simulink library "lib_controller"  (R2015a)
settings: Solver=ode45  StartTime=0.0  StopTime=10.0  RelTol=1e-3
values from neighbouring files (symbols this model uses):
  CG_0 = [0,0,0.02]'    [SetupComplete.m]
  g = 9.81    [SetupComplete.m]
  h_M = 0.064    [SetupComplete.m]
  I_BAC_0 = [ Ix,0,Ixz;0,Iy,0;Ixz,0,Iz]    [SetupComplete.m]
  l = 0.3450    (= 0.345)    [NDI_components.m]    (also in SetupComplete.m; robust_controller.m)
  m = 3.51    [SetupComplete.m]
  m_0 = 2.61    [SetupComplete.m]
  m_M = 0.300    (= 0.3)    [SetupComplete.m]
  T_sim = 0.01    [Run3Copter.m]
undefined symbols (not defined in the file or in its folder): Theta_1_roll_last, Theta_2_roll_last, Theta_3_roll_last, V_long_lastA_w_z, V_long_lastAoA, V_roll_last, V_yaw_last, W_long_lastA_w_z, W_long_lastAoA, W_roll_last, W_yaw_last
libraries: simulink x65, Adaptive_FaultTolerantControl x8, lib_controller x5, qcatlib x4, dspinverses x4, aerolibtransform2 x3, aerolib6dofsys x1
(part 1 of 10)
settings Model: Creator=juan  LastModifiedBy=juan

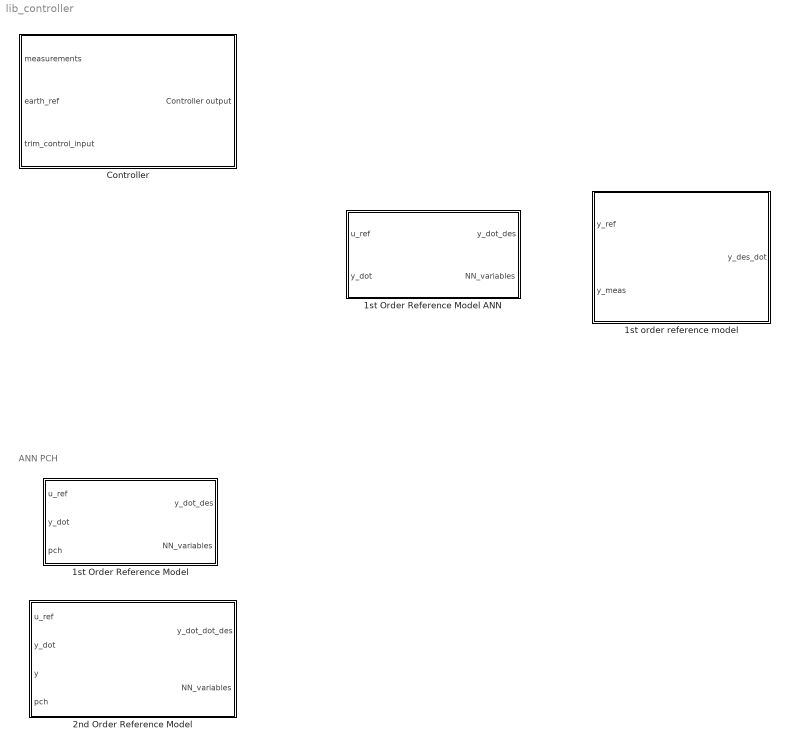
== system lib_controller ==
  note: ANN PCH
  1st Order Reference Model : Subsystem  mask{tau=0.25, r=1}
      mask prompts: tau "Time Constant"; r "NN Error dynamic ratio"
      mask help:
      | 1st Order Model Reference System
      | Tau is the time constant and sets the dynamics of the reference model.
      | Error dynamic ratio sets how faster compared to the reference model is the
      | NN output going to try to compensate for the inversion error.
      mask Display:
      | K_ref=1/tau;
      | TF = tf([K_ref],[1 K_ref]);
      | 
      | [y,t]=step(TF);
      | S = stepinfo(y,t);
      | 
      | pos = get_param(gcb, 'Position');
      | width = pos(3) - pos(1);
      | height = pos(4) - pos(2);
      | t = t.*width/max(t);
      | y=y.*height/max(y);
      | plot(t,y);
      | S2 = stepinfo(y,t);
      | 
      | if S.Overshoot==0 % 1st order response
      |     text(S2.RiseTime ,height*0.85,['Rise time = ',num2str(S.RiseTime),'s' ]);
      |     text(S2.RiseTime ,height*0.75,['Settling Time = ',num2str(S.SettlingTime)]);
      | 
      | elseif S.Overshoot<0.05 % 2nd order response
      |     text(width*0.5 ,height*0.9,['Rise time = ',num2str(S.RiseTime),'s' ]);
      |     text(width*0.5 ,height*0.8,['Pike time = ',num2str(S.PeakTime),'s' ]);
      |     text(width*0.5 ,height*0.7,['Os = ',num2str(S.Peak)]);
      |     text(width*0.5 ,height*0.6,['SettlingTime = ',num2str(S.SettlingTime)]);
      | else % 2nd order response
      |     text(S2.PeakTime ,S2.Peak*0.85,['Peak time = ',num2str(S.PeakTime),'s' ]);
      |     text(S2.PeakTime ,S2.Peak*0.75,['Os = ',num2str(S.Peak)]);
      |     text(S2.PeakTime ,S2.Peak*0.65,['SettlingTime = ',num2str(S.SettlingTime)]);
      | end
      | 
      | 
      | [num,den] = tfdata(TF);
      | dpoly(num{:},den{:}, 's');
  1st Order Reference Model ANN : Subsystem  mask{tau=0.25, r=1}
      mask prompts: tau "Time Constant"; r "NN Error dynamic ratio"
      mask help:
      | 1st Order Model Reference System
      | Tau is the time constant and sets the dynamics of the reference model.
      | Error dynamic ratio sets how faster compared to the reference model is the
      | NN output going to try to compensate for the inversion error.
      mask Display:
      | K_ref=1/tau;
      | TF = tf([K_ref],[1 K_ref]);
      | 
      | [y,t]=step(TF);
      | S = stepinfo(y,t);
      | 
      | pos = get_param(gcb, 'Position');
      | width = pos(3) - pos(1);
      | height = pos(4) - pos(2);
      | t = t.*width/max(t);
      | y=y.*height/max(y);
      | plot(t,y);
      | S2 = stepinfo(y,t);
      | 
      | if S.Overshoot==0 % 1st order response
      |     text(S2.RiseTime ,height*0.85,['Rise time = ',num2str(S.RiseTime),'s' ]);
      |     text(S2.RiseTime ,height*0.75,['Settling Time = ',num2str(S.SettlingTime)]);
      | 
      | elseif S.Overshoot<0.05 % 2nd order response
      |     text(width*0.5 ,height*0.9,['Rise time = ',num2str(S.RiseTime),'s' ]);
      |     text(width*0.5 ,height*0.8,['Pike time = ',num2str(S.PeakTime),'s' ]);
      |     text(width*0.5 ,height*0.7,['Os = ',num2str(S.Peak)]);
      |     text(width*0.5 ,height*0.6,['SettlingTime = ',num2str(S.SettlingTime)]);
      | else % 2nd order response
      |     text(S2.PeakTime ,S2.Peak*0.85,['Peak time = ',num2str(S.PeakTime),'s' ]);
      |     text(S2.PeakTime ,S2.Peak*0.75,['Os = ',num2str(S.Peak)]);
      |     text(S2.PeakTime ,S2.Peak*0.65,['SettlingTime = ',num2str(S.SettlingTime)]);
      | end
      | 
      | 
      | [num,den] = tfdata(TF);
      | dpoly(num{:},den{:}, 's');
  1st order reference model : Subsystem  mask(1st order model reference block){Kref=10, Kb=10, fi=0.25, fc=0.5, Kf=1}
      mask prompts: Kref "1st order reference gain"; Kb "Bandwidth gain"; fi "Integral gain"; fc "Command FF gain"; Kf "Command_dot FF gain"
      mask help:
      | Generates a desired first order derivative of a commanded output taking
      | into account the current measured output.
      | Kref is the gain that determines the first order system between y_ref and
      | y_commanded signals. Ycom/Yref = Kref/(1 + Kref)
      | fi and fc can be defaulted to 0.25 and 0.5 for a critically damped 2nd
      | order response between y_meas and the error signal (y_com - y_meas) considering
      | a perfect dynamic inversion.
      mask Help:
      | Juan Herrero Macias <jn.herrerom@gmail.com>
      | This architecture can be found and explained in Fault-tolerant Flight
      | Control and Guidance Systems, Ducard, Guillaume.
      mask TypeOptions Kref: Kref gain/Gain
      mask TypeOptions Kb: Bandwidth gain/Gain
      mask TypeOptions fi: Integral gain/Gain
      mask TypeOptions fc: Command FF gain/Gain
      mask TypeOptions Kf: Command_dot FF gain/Gain
  2nd Order Reference Model : Subsystem  mask{omega_n=4, xi=1.1, r=0}
      mask prompts: omega_n "Natural Frequency"; xi "Damping"; r "NN Error dynamic ratio"
      mask help:
      | 2nd Order Model Reference System
      | Natural frequency and damping ratio set the dynamic of the model reference.
      | Error dynamic ratio sets how faster compared to the reference model dynamics
      | is the settling time of the inversion error provided by the NN.
      mask Display:
      | TF = tf([omega_n^2],[1 2*xi*omega_n omega_n^2]);
      | 
      | [y,t]=step(TF);
      | S = stepinfo(y,t);
      | 
      | pos = get_param(gcb, 'Position');
      | width = pos(3) - pos(1);
      | height = pos(4) - pos(2);
      | t = t.*width/max(t);
      | y=y.*height/max(y);
      | plot(t,y);
      | S2 = stepinfo(y,t);
      | 
      | if S.Overshoot==0 % 1st order response
      |     text(S2.RiseTime ,height*0.85,['Rise time = ',num2str(S.RiseTime),'s' ]);
      |     text(S2.RiseTime ,height*0.75,['Settling Time = ',num2str(S.SettlingTime)]);
      | 
      | elseif S.Overshoot<0.05 % 2nd order response
      |     text(width*0.5 ,height*0.9,['Rise time = ',num2str(S.RiseTime),'s' ]);
      |     text(width*0.5 ,height*0.8,['Pike time = ',num2str(S.PeakTime),'s' ]);
      |     text(width*0.5 ,height*0.7,['Os = ',num2str(S.Peak)]);
      |     text(width*0.5 ,height*0.6,['SettlingTime = ',num2str(S.SettlingTime)]);
      | else % 2nd order response
      |     text(S2.PeakTime ,S2.Peak*0.85,['Peak time = ',num2str(S.PeakTime),'s' ]);
      |     text(S2.PeakTime ,S2.Peak*0.75,['Os = ',num2str(S.Peak)]);
      |     text(S2.PeakTime ,S2.Peak*0.65,['SettlingTime = ',num2str(S.SettlingTime)]);
      | end
      | 
      | 
      | [num,den] = tfdata(TF);
      | dpoly(num{:},den{:}, 's');
  Controller : Subsystem  Variant=on  OverrideUsingVariant=Variant1

== system lib_controller/1st Order Reference Model ==
  u_ref : Inport
  y_dot : Inport  Port=2
  pch : Inport  Port=3
  A_error_dynamics : Constant  Value=-r/tau
  Bus Creator : BusCreator  Inputs=6
  Kp_y : Gain  Gain=r/tau
  P_error_dynamics : Constant  Value=tau/r
  Reference Model : Subsystem  mask{tau=tau, y_i=0}
      mask prompts: tau "1st order time constant (tau)"; y_i "Initial state"
      mask init:
      | K_ref=1/tau;
      mask Display:
      | K_ref=1/tau;
      | TF = tf([K_ref],[1 K_ref]);
      | 
      | [y,t]=step(TF);
      | S = stepinfo(y,t);
      | 
      | pos = get_param(gcb, 'Position');
      | width = pos(3) - pos(1);
      | height = pos(4) - pos(2);
      | t = t.*width/max(t);
      | y=y.*height/max(y);
      | plot(t,y);
      | S2 = stepinfo(y,t);
      | 
      | if S.Overshoot==0 % 1st order response
      |     text(S2.RiseTime ,height*0.85,['Rise time = ',num2str(S.RiseTime),'s' ]);
      |     text(S2.RiseTime ,height*0.75,['Settling Time = ',num2str(S.SettlingTime)]);
      | 
      | elseif S.Overshoot<0.05 % 2nd order response
      |     text(width*0.5 ,height*0.9,['Rise time = ',num2str(S.RiseTime),'s' ]);
      |     text(width*0.5 ,height*0.8,['Pike time = ',num2str(S.PeakTime),'s' ]);
      |     text(width*0.5 ,height*0.7,['Os = ',num2str(S.Peak)]);
      |     text(width*0.5 ,height*0.6,['SettlingTime = ',num2str(S.SettlingTime)]);
      | else % 2nd order response
      |     text(S2.PeakTime ,S2.Peak*0.85,['Peak time = ',num2str(S.PeakTime),'s' ]);
      |     text(S2.PeakTime ,S2.Peak*0.75,['Os = ',num2str(S.Peak)]);
      |     text(S2.PeakTime ,S2.Peak*0.65,['SettlingTime = ',num2str(S.SettlingTime)]);
      | end
      | 
      | 
      | [num,den] = tfdata(TF);
      | dpoly(num{:},den{:}, 's');
  Sum17 : Sum  Inputs=++|
  Sum22 : Sum  Inputs=|+-
  b_error_dynamics : Constant  Value=[1]  VectorParams1D=off
  y_dot_des : Outport
  NN_variables : Outport  Port=2
  wires:
  u_ref/1 -> Reference Model/1(u)
  Reference Model/2(y) -> Bus Creator/2, Sum22/1  "y_c"
  Reference Model/1(y_dot) -> Bus Creator/3, Sum17/1  "y_dot_c"
  y_dot/1 -> Sum22/2
  Sum22/1 -> Bus Creator/1, Kp_y/1  "y_error"
  Kp_y/1 -> Sum17/2
  Sum17/1 -> y_dot_des/1
  Bus Creator/1 -> NN_variables/1
  A_error_dynamics/1 -> Bus Creator/5  "A_error_dyn"
  P_error_dynamics/1 -> Bus Creator/4  "P_error_dyn"
  b_error_dynamics/1 -> Bus Creator/6  "b_error_dyn"
  pch/1 -> Reference Model/2(pch)

== system lib_controller/1st Order Reference Model ANN ==
  u_ref : Inport
  y_dot : Inport  Port=2
  A_error_dynamics : Constant  Value=-r/tau
  Bus Creator : BusCreator  Inputs=6
  Kp_y : Gain  Gain=r/tau
  P_error_dynamics : Constant  Value=tau/r
  Reference Model : Subsystem  mask{tau=tau, y_i=0}
      mask prompts: tau "1st order time constant (tau)"; y_i "Initial state"
      mask init:
      | K_ref=1/tau;
      mask Display:
      | K_ref=1/tau;
      | TF = tf([K_ref],[1 K_ref]);
      | 
      | [y,t]=step(TF);
      | S = stepinfo(y,t);
      | 
      | pos = get_param(gcb, 'Position');
      | width = pos(3) - pos(1);
      | height = pos(4) - pos(2);
      | t = t.*width/max(t);
      | y=y.*height/max(y);
      | plot(t,y);
      | S2 = stepinfo(y,t);
      | 
      | if S.Overshoot==0 % 1st order response
      |     text(S2.RiseTime ,height*0.85,['Rise time = ',num2str(S.RiseTime),'s' ]);
      |     text(S2.RiseTime ,height*0.75,['Settling Time = ',num2str(S.SettlingTime)]);
      | 
      | elseif S.Overshoot<0.05 % 2nd order response
      |     text(width*0.5 ,height*0.9,['Rise time = ',num2str(S.RiseTime),'s' ]);
      |     text(width*0.5 ,height*0.8,['Pike time = ',num2str(S.PeakTime),'s' ]);
      |     text(width*0.5 ,height*0.7,['Os = ',num2str(S.Peak)]);
      |     text(width*0.5 ,height*0.6,['SettlingTime = ',num2str(S.SettlingTime)]);
      | else % 2nd order response
      |     text(S2.PeakTime ,S2.Peak*0.85,['Peak time = ',num2str(S.PeakTime),'s' ]);
      |     text(S2.PeakTime ,S2.Peak*0.75,['Os = ',num2str(S.Peak)]);
      |     text(S2.PeakTime ,S2.Peak*0.65,['SettlingTime = ',num2str(S.SettlingTime)]);
      | end
      | 
      | 
      | [num,den] = tfdata(TF);
      | dpoly(num{:},den{:}, 's');
  Sum17 : Sum  Inputs=++|
  Sum22 : Sum  Inputs=|+-
  b_error_dynamics : Constant  Value=[1]  VectorParams1D=off
  y_dot_des : Outport
  NN_variables : Outport  Port=2
  wires:
  b_error_dynamics/1 -> Bus Creator/6  "b_error_dyn"
  P_error_dynamics/1 -> Bus Creator/4  "P_error_dyn"
  A_error_dynamics/1 -> Bus Creator/5  "A_error_dyn"
  Bus Creator/1 -> NN_variables/1
  Sum17/1 -> y_dot_des/1
  Kp_y/1 -> Sum17/2
  Sum22/1 -> Kp_y/1, Bus Creator/1  "y_error"
  y_dot/1 -> Sum22/2
  Reference Model/1(y_dot) -> Sum17/1, Bus Creator/3  "y_dot_c"
  Reference Model/2(y) -> Sum22/1, Bus Creator/2  "y_c"
  u_ref/1 -> Reference Model/1(u)

== system lib_controller/1st order reference model ==
  y_ref : Inport
  y_meas : Inport  Port=2
  Bandwidth gain : Gain  Gain=Kb
  Bandwidth gain 1 : Gain  Gain=Kb
  Command FF gain : Gain  Gain=fc
  Command_dot FF gain : Gain  Gain=Kf
  Integral gain : Gain  Gain=fi
  Integrator : Integrator
  Integrator1 : Integrator
  Kref gain : Gain  Gain=Kref
  Sum15 : Sum  Inputs=|+-
  Sum16 : Sum  Inputs=++-
  Sum17 : Sum  Inputs=++|
  Sum5 : Sum  Inputs=|+-
  y_des_dot : Outport
  wires:
  Sum5/1 -> Kref gain/1
  Sum15/1 -> Bandwidth gain 1/1
  Bandwidth gain/1 -> Sum17/2
  Sum17/1 -> y_des_dot/1
  Integrator1/1 -> Sum16/2
  Kref gain/1 -> Command_dot FF gain/1, Integrator/1  "y_dot_c"
  Sum16/1 -> Bandwidth gain/1
  y_meas/1 -> Sum15/2, Sum16/3
  Integrator/1 -> Sum5/2, Sum15/1, Command FF gain/1  "y_c"
  Command FF gain/1 -> Sum16/1
  Command_dot FF gain/1 -> Sum17/1
  y_ref/1 -> Sum5/1
  Bandwidth gain 1/1 -> Integral gain/1
  Integral gain/1 -> Integrator1/1

== system lib_controller/2nd Order Reference Model ==
  u_ref : Inport
  y_dot : Inport  Port=2
  y : Inport  Port=3
  pch : Inport  Port=4
  A_error_dynamics1 : Constant  Value=[0, 1; -(r*omega_n)^2, -2*xi*(r*omega_n)]
  Bus Creator : BusCreator  Inputs=8
  Kd_y_dot : Gain  Gain=2*xi*(r*omega_n)
  Kp_y : Gain  Gain=(r*omega_n)^2
  P_error_dynamics1 : Constant  Value=[((r*omega_n)^2+1)/(2*xi*(r*omega_n)) + 2*xi*(r*omega_n)/(r*omega_n)^2, 1/(r*omega_n)^2; 1/(r*omega_n)^2, (1+1/(r*omega_n)^2)/(2*xi*(r*omega_n))]
  Reference Model1 : Subsystem  mask{omega_n=omega_n, xi=xi}
      mask prompts: omega_n "Natural Frequency"; xi "Damping"
      mask help:
      | 2nd Order System
      | Only provides output acceleration
      mask Display:
      | TF = tf([omega_n^2],[1 xi*omega_n omega_n^2]);
      | 
      | [y,t]=step(TF);
      | S = stepinfo(y,t);
      | 
      | pos = get_param(gcb, 'Position');
      | width = pos(3) - pos(1);
      | height = pos(4) - pos(2);
      | t = t.*width/max(t);
      | y=y.*height/max(y);
      | plot(t,y);
      | S2 = stepinfo(y,t);
      | 
      | if S.Overshoot==0 % 1st order response
      |     text(S2.RiseTime ,height*0.85,['Rise time = ',num2str(S.RiseTime),'s' ]);
      |     text(S2.RiseTime ,height*0.75,['Settling Time = ',num2str(S.SettlingTime)]);
      | 
      | elseif S.Overshoot<0.05 % 2nd order response
      |     text(width*0.5 ,height*0.9,['Rise time = ',num2str(S.RiseTime),'s' ]);
      |     text(width*0.5 ,height*0.8,['Pike time = ',num2str(S.PeakTime),'s' ]);
      |     text(width*0.5 ,height*0.7,['Os = ',num2str(S.Peak)]);
      |     text(width*0.5 ,height*0.6,['SettlingTime = ',num2str(S.SettlingTime)]);
      | else % 2nd order response
      |     text(S2.PeakTime ,S2.Peak*0.85,['Peak time = ',num2str(S.PeakTime),'s' ]);
      |     text(S2.PeakTime ,S2.Peak*0.75,['Os = ',num2str(S.Peak)]);
      |     text(S2.PeakTime ,S2.Peak*0.65,['SettlingTime = ',num2str(S.SettlingTime)]);
      | end
      | 
      | 
      | [num,den] = tfdata(TF);
      | dpoly(num{:},den{:}, 's');
  Sum19 : Sum  Inputs=|+-
  Sum20 : Sum  Inputs=+++
  Sum21 : Sum  Inputs=|+-
  b_error_dynamics : Constant  Value=[0; 1]  VectorParams1D=off
  y_dot_dot_des : Outport
  NN_variables : Outport  Port=2
  wires:
  Reference Model1/1(y_dot_dot) -> Bus Creator/5, Sum20/1  "y_dot_dot_c"
  Reference Model1/3(y) -> Bus Creator/3, Sum19/1  "y_c"
  u_ref/1 -> Reference Model1/1(u)
  y/1 -> Sum19/2
  Sum19/1 -> Bus Creator/1, Kp_y/1  "y_error"
  Reference Model1/2(y_dot) -> Bus Creator/4, Sum21/1  "y_dot_c"
  y_dot/1 -> Sum21/2
  Sum21/1 -> Kd_y_dot/1, Bus Creator/2  "y_dot_error"
  Kp_y/1 -> Sum20/3
  Kd_y_dot/1 -> Sum20/2
  Sum20/1 -> y_dot_dot_des/1
  Bus Creator/1 -> NN_variables/1
  P_error_dynamics1/1 -> Bus Creator/6  "P_error_dyn"
  A_error_dynamics1/1 -> Bus Creator/7  "A_error_dyn"
  b_error_dynamics/1 -> Bus Creator/8  "b_error_dyn"
  pch/1 -> Reference Model1/2(pch)

== system lib_controller/Controller ==
  note: Controller output:
      | Throttle [%]
      | Actuator angle [deg]
  note: Controller output:
      | 1. tau_1 [0-1] (Thr ottle motor 1)
      | 2. eta_1 (deg)  (Pan arm 1)
      | 3. gamma_1 (deg)  (Tilt arm 1)
      |
      | 4. tau_2 [0-1] (Throttle motor 2)
      | 5. eta_2 (deg)  (Pan arm 2)
      | 6. gamma_2 (deg)  (Tilt arm 2)
      |
      | 7. tau_3 [0-1] (Throttle motor 3)
      | 8. eta_3 (deg)  (Pan arm  3)
      | 9. gamma_3 (deg)  (Tilt arm 3)
  measurements : Inport
  earth_ref : Inport  Port=2
  trim_control_input : Inport  Port=3
  4DOF PID Controller : Subsystem  Variant=on  VariantControl=(default)  OverrideUsingVariant=Variant3
  NDI+CA Controller : Subsystem  Variant=on  VariantControl=Variant1  OverrideUsingVariant=Variant6
  Controller output : Outport

== system lib_controller/1st Order Reference Model/Reference Model ==
  u : Inport
  pch : Inport  Port=2
  Add : Sum  Inputs=|+-
  Add1 : Sum  Inputs=++|
  Integrator : Integrator
  K_ref : Gain  Gain=K_ref
  y_dot : Outport
  y : Outport  Port=2
  wires:
  Integrator/1 -> Add/2, y/1
  Add/1 -> K_ref/1
  u/1 -> Add/1
  K_ref/1 -> Add1/2
  Add1/1 -> y_dot/1, Integrator/1
  pch/1 -> Add1/1

== system lib_controller/1st Order Reference Model ANN/Reference Model ==
  u : Inport
  Add : Sum  Inputs=|+-
  Integrator : Integrator
  K_ref : Gain  Gain=K_ref
  y_dot : Outport
  y : Outport  Port=2
  wires:
  K_ref/1 -> Integrator/1, y_dot/1
  u/1 -> Add/1
  Add/1 -> K_ref/1
  Integrator/1 -> y/1, Add/2

== system lib_controller/2nd Order Reference Model/Reference Model1 ==
  u : Inport
  pch : Inport  Port=2
  Add : Sum  Inputs=|+-
  Add1 : Sum  Inputs=++-
  Integrator : Integrator
  Integrator1 : Integrator
  K_ref1 : Gain  Gain=2*xi*omega_n
  K_ref3 : Gain  Gain=omega_n^2
  y_dot_dot : Outport
  y_dot : Outport  Port=2
  y : Outport  Port=3
  wires:
  Integrator1/1 -> Integrator/1, K_ref1/1, y_dot/1
  Integrator/1 -> y/1, Add/2
  u/1 -> Add/1
  Add/1 -> K_ref3/1
  Add1/1 -> y_dot_dot/1, Integrator1/1  "y_dot_dot"
  K_ref3/1 -> Add1/2
  K_ref1/1 -> Add1/3
  pch/1 -> Add1/1

== system lib_controller/Controller/4DOF PID Controller ==
  measurements : Inport
  earth_ref : Inport  Port=2
  trim_control_input : Inport  Port=3
  4DOF PI Angle Controller : Subsystem  VariantControl=Variant1
  4DOF PI Angle Trimming Controller : Subsystem  VariantControl=Variant4
  4DOF PI Rate Trimming Controller : Subsystem  VariantControl=Variant2
  4DOF PID Speed Controller : Subsystem  VariantControl=Variant3
  Controller output : Outport

== system lib_controller/Controller/NDI+CA Controller ==
  note: 4 DOF
  note: 9 DOF
  measurements : Inport
  earth_ref : Inport  Port=2
  trim_control_input : Inport  Port=3
  " 9DOF NDI+CA Controller - No massic update" : Subsystem  VariantControl=Variant2
  4DOF ANN+NDI+CA Controller - No massic update : Subsystem  VariantControl=Variant4
  4DOF NDI+CA Controller : Subsystem  VariantControl=Variant3
  4DOF NDI+CA Controller - No massic update : Subsystem  VariantControl=Variant5
  9DOF ANN+NDI+CA Controller - No massic update : Subsystem  VariantControl=Variant6
  9DOF NDI+CA Controller : Subsystem  VariantControl=(default)
  Controller output : Outport

== system lib_controller/Controller/4DOF PID Controller/4DOF PI Angle Controller ==
  note: This DCM is Tb->e
      | Xbody = DCM x Xearth
  note: Proportional controller around the hovering point. Body rates will be very similar to euler rates.
  note: INNER RATE LOOP TUNING
  note: INNER ANGLE LOOP TUNING
  measurements : Inport
  earth_ref : Inport  Port=2
  trim_control_input : Inport  Port=3
  Bus Selector : BusSelector  OutputSignals=euler,euler_dot,X_e,DCM,V_b
  Demux{,1,3..8} (8 alike) : Demux  Outputs=3
  Earth to body : Product  Multiplication=Matrix(*)
  Inner Rate Controller1 : ModelReference  ModelNameDialog=Inner_Rate_Controller  SimulationMode=Normal  ModelReferenceVersion=1.1241  CopyOfModelName=Inner_Rate_Controller
  Mux1 : Mux  Inputs=3
  Mux2 : Mux  Inputs=3
  Mux3 : Mux  Inputs=3
  PID Controller : simulink/Continuous/PID Controller  Controller=PI  TimeDomain=Continuous-time  SampleTime=-1  IntegratorMethod=Forward Euler  FilterMethod=Forward Euler  Form=Parallel  UseFilter=on  ControllerParametersSource=internal  P=1  I=1  D=0  N=100  InitialConditionSource=internal  InitialConditionForIntegrator=0  InitialConditionForFilter=0  ExternalReset=none  LimitOutput=off  UpperSaturationLimit=inf  LowerSaturationLimit=-inf  LinearizeAsGain=on  AntiWindupMode=none  Kb=1  TrackingMode=off  Kt=1  PParamMin=[]  PParamMax=[]  IParamMin=[]  IParamMax=[]  DParamMin=[]  DParamMax=[]  NParamMin=[]  NParamMax=[]  KbParamMin=[]  KbParamMax=[]  KtParamMin=[]  KtParamMax=[]  POutMin=[]  POutMax=[]  IOutMin=[]  IOutMax=[]  DOutMin=[]  DOutMax=[]  NOutMin=[]  NOutMax=[]  KbOutMin=[]  KbOutMax=[]  KtOutMin=[]  KtOutMax=[]  IntegratorOutMin=[]  IntegratorOutMax=[]  FilterOutMin=[]  FilterOutMax=[]  SumOutMin=[]  SumOutMax=[]  SumI1OutMin=[]  SumI1OutMax=[]  SumI2OutMin=[]  SumI2OutMax=[]  SumI3OutMin=[]  SumI3OutMax=[]  SumDOutMin=[]  SumDOutMax=[]  SaturationOutMin=[]  SaturationOutMax=[]  IntegratorContinuousStateAttributes=''  IntegratorStateMustResolveToSignalObject=off  IntegratorRTWStateStorageClass=Auto  FilterContinuousStateAttributes=''  FilterStateMustResolveToSignalObject=off  FilterRTWStateStorageClass=Auto  DifferentiatorICPrevScaledInput=0  DifferentiatorOutMin=[]  DifferentiatorOutMax=[]
  PID Controller1 : simulink/Continuous/PID Controller  Controller=PI  TimeDomain=Continuous-time  SampleTime=-1  IntegratorMethod=Forward Euler  FilterMethod=Forward Euler  Form=Parallel  UseFilter=on  ControllerParametersSource=internal  P=1  I=1  D=0  N=100  InitialConditionSource=internal  InitialConditionForIntegrator=0  InitialConditionForFilter=0  ExternalReset=none  LimitOutput=off  UpperSaturationLimit=inf  LowerSaturationLimit=-inf  LinearizeAsGain=on  AntiWindupMode=none  Kb=1  TrackingMode=off  Kt=1  PParamMin=[]  PParamMax=[]  IParamMin=[]  IParamMax=[]  DParamMin=[]  DParamMax=[]  NParamMin=[]  NParamMax=[]  KbParamMin=[]  KbParamMax=[]  KtParamMin=[]  KtParamMax=[]  POutMin=[]  POutMax=[]  IOutMin=[]  IOutMax=[]  DOutMin=[]  DOutMax=[]  NOutMin=[]  NOutMax=[]  KbOutMin=[]  KbOutMax=[]  KtOutMin=[]  KtOutMax=[]  IntegratorOutMin=[]  IntegratorOutMax=[]  FilterOutMin=[]  FilterOutMax=[]  SumOutMin=[]  SumOutMax=[]  SumI1OutMin=[]  SumI1OutMax=[]  SumI2OutMin=[]  SumI2OutMax=[]  SumI3OutMin=[]  SumI3OutMax=[]  SumDOutMin=[]  SumDOutMax=[]  SaturationOutMin=[]  SaturationOutMax=[]  IntegratorContinuousStateAttributes=''  IntegratorStateMustResolveToSignalObject=off  IntegratorRTWStateStorageClass=Auto  FilterContinuousStateAttributes=''  FilterStateMustResolveToSignalObject=off  FilterRTWStateStorageClass=Auto  DifferentiatorICPrevScaledInput=0  DifferentiatorOutMin=[]  DifferentiatorOutMax=[]
  PID Controller2 : simulink/Continuous/PID Controller  Controller=PI  TimeDomain=Continuous-time  SampleTime=-1  IntegratorMethod=Forward Euler  FilterMethod=Forward Euler  Form=Parallel  UseFilter=on  ControllerParametersSource=internal  P=1  I=0.1  D=0  N=100  InitialConditionSource=internal  InitialConditionForIntegrator=0  InitialConditionForFilter=0  ExternalReset=none  LimitOutput=off  UpperSaturationLimit=inf  LowerSaturationLimit=-inf  LinearizeAsGain=on  AntiWindupMode=none  Kb=1  TrackingMode=off  Kt=1  PParamMin=[]  PParamMax=[]  IParamMin=[]  IParamMax=[]  DParamMin=[]  DParamMax=[]  NParamMin=[]  NParamMax=[]  KbParamMin=[]  KbParamMax=[]  KtParamMin=[]  KtParamMax=[]  POutMin=[]  POutMax=[]  IOutMin=[]  IOutMax=[]  DOutMin=[]  DOutMax=[]  NOutMin=[]  NOutMax=[]  KbOutMin=[]  KbOutMax=[]  KtOutMin=[]  KtOutMax=[]  IntegratorOutMin=[]  IntegratorOutMax=[]  FilterOutMin=[]  FilterOutMax=[]  SumOutMin=[]  SumOutMax=[]  SumI1OutMin=[]  SumI1OutMax=[]  SumI2OutMin=[]  SumI2OutMax=[]  SumI3OutMin=[]  SumI3OutMax=[]  SumDOutMin=[]  SumDOutMax=[]  SaturationOutMin=[]  SaturationOutMax=[]  IntegratorContinuousStateAttributes=''  IntegratorStateMustResolveToSignalObject=off  IntegratorRTWStateStorageClass=Auto  FilterContinuousStateAttributes=''  FilterStateMustResolveToSignalObject=off  FilterRTWStateStorageClass=Auto  DifferentiatorICPrevScaledInput=0  DifferentiatorOutMin=[]  DifferentiatorOutMax=[]
  Sum : Sum  Inputs=|+-
  Sum1 : Sum  Inputs=-+|
  Sum2 : Sum  Inputs=|++
  Sum3 : Sum  Inputs=-+|
  Sum4 : Sum  Inputs=|+-
  euler_ref : Constant  Value=[0,0,0]
  Controller output : Outport
  wires:
  [psi_error] -> PID Controller2/1
  [theta_error] -> PID Controller1/1
  PID Controller2/1 -> [r_ref]
  PID Controller1/1 -> [q_ref]
  PID Controller/1 -> [p_ref]
  [phi_error] -> PID Controller/1
  Demux3/3 -> [r]
  Demux3/2 -> [q]
  Demux3/1 -> [p]
  measurements/1 -> Bus Selector/1
  Sum2/1 -> Controller output/1
  Bus Selector/2 -> Demux3/1, Sum1/1  "<euler_dot>"
  Sum1/1 -> Demux/1
  Demux/3 -> [r_error]
  Demux/2 -> [q_error]
  Demux/1 -> [p_error]
  trim_control_input/1 -> [trimmed_input]
  [trimmed_input] -> Sum2/2
  Mux2/1 -> Sum1/2
  [q_ref] -> Mux2/2
  [p_ref] -> Mux2/1
  [r_ref] -> Mux2/3
  Inner Rate Controller1/1 -> Sum2/1
  [p_error] -> Inner Rate Controller1/1
  [q_error] -> Inner Rate Controller1/2
  [r_error] -> Inner Rate Controller1/3
  Bus Selector/3 -> Demux5/1, Sum3/1  "<X_e>"
  Demux5/3 -> [Z_earth]
  Demux5/2 -> [Y_earth]
  Demux5/1 -> [X_earth]
  Demux4/3 -> [z_error]
  Demux4/2 -> [y_error]
  Demux4/1 -> [x_error]
  Mux1/1 -> Sum3/2
  [Yearth_ref] -> Mux1/2
  [Xearth_ref] -> Mux1/1
  [Zearth_ref] -> Mux1/3
  Mux3/1 -> Sum4/1
  Demux7/1 -> [vx_b]
  Demux7/2 -> [vy_b]
  Demux7/3 -> [vz_b]
  Bus Selector/5 -> Demux7/1, Sum4/2  "<V_b>"
  Sum4/1 -> Demux6/1
  Demux6/1 -> [vx_error]
  Demux6/2 -> [vy_error]
  Demux6/3 -> [vz_error]
  [Vy_body_ref] -> Mux3/2
  [Vx_body_ref] -> Mux3/1
  [Vz_body_ref] -> Mux3/3
  Bus Selector/4 -> Earth to body/2  "<DCM>"
  Earth to body/1 -> Demux4/1
  Sum3/1 -> Earth to body/1
  Demux8/3 -> [Zearth_ref]
  Demux8/2 -> [Yearth_ref]
  Demux8/1 -> [Xearth_ref]
  earth_ref/1 -> Demux8/1
  Bus Selector/1 -> Sum/2  "<euler>"
  Sum/1 -> Demux1/1
  Demux1/1 -> [phi_error]
  Demux1/2 -> [theta_error]
  Demux1/3 -> [psi_error]
  euler_ref/1 -> Sum/1

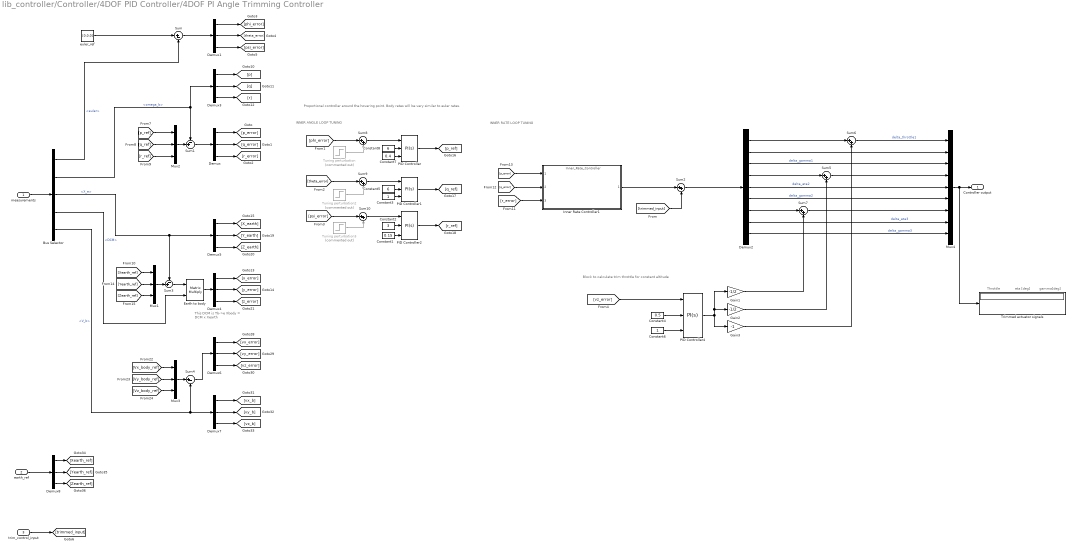
== system lib_controller/Controller/4DOF PID Controller/4DOF PI Angle Trimming Controller ==
  note: Throttle
  note: Block to calculate trim throttle for constant altitude
  note: INNER ANGLE LOOP TUNING
  note: INNER RATE LOOP TUNING
  note: Proportional controller around the hovering point. Body rates will be very similar to euler rates.
  note: This DCM is Tb->e
      | Xbody = DCM x Xearth
  note: eta [deg]
  note: gamma[deg]
  measurements : Inport
  earth_ref : Inport  Port=2
  trim_control_input : Inport  Port=3
  Bus Selector : BusSelector  OutputSignals=euler,omega_b,X_e,DCM,V_b
  Constant1 : Constant  Value=0.15
  Constant2 : Constant  Value=3
  Constant3 : Constant
  Constant4 : Constant  Value=0.5
  Constant5 : Constant  Value=6
  Constant6 : Constant
  Constant7 : Constant  Value=0.4
  Constant8 : Constant  Value=6
  Demux{,1,3..8} (8 alike) : Demux  Outputs=3
  Demux2 : Demux  Outputs=9
  Earth to body : Product  Multiplication=Matrix(*)
  Gain1 : Gain  Gain=-1/2
  Gain2 : Gain  Gain=-1/2
  Gain3 : Gain  Gain=-1
  Inner Rate Controller1 : ModelReference  ModelNameDialog=Inner_Rate_Controller  SimulationMode=Normal  ModelReferenceVersion=1.1241  CopyOfModelName=Inner_Rate_Controller
  Mux1 : Mux  Inputs=3
  Mux2 : Mux  Inputs=3
  Mux3 : Mux  Inputs=3
  Mux4 : Mux  Inputs=9
  PID Controller : simulink/Continuous/PID Controller  Controller=PI  TimeDomain=Continuous-time  SampleTime=-1  IntegratorMethod=Forward Euler  FilterMethod=Forward Euler  Form=Parallel  UseFilter=on  ControllerParametersSource=external  P=1  I=1  D=0  N=100  InitialConditionSource=internal  InitialConditionForIntegrator=0  InitialConditionForFilter=0  ExternalReset=none  LimitOutput=off  UpperSaturationLimit=inf  LowerSaturationLimit=-inf  LinearizeAsGain=on  AntiWindupMode=none  Kb=1  TrackingMode=off  Kt=1  PParamMin=[]  PParamMax=[]  IParamMin=[]  IParamMax=[]  DParamMin=[]  DParamMax=[]  NParamMin=[]  NParamMax=[]  KbParamMin=[]  KbParamMax=[]  KtParamMin=[]  KtParamMax=[]  POutMin=[]  POutMax=[]  IOutMin=[]  IOutMax=[]  DOutMin=[]  DOutMax=[]  NOutMin=[]  NOutMax=[]  KbOutMin=[]  KbOutMax=[]  KtOutMin=[]  KtOutMax=[]  IntegratorOutMin=[]  IntegratorOutMax=[]  FilterOutMin=[]  FilterOutMax=[]  SumOutMin=[]  SumOutMax=[]  SumI1OutMin=[]  SumI1OutMax=[]  SumI2OutMin=[]  SumI2OutMax=[]  SumI3OutMin=[]  SumI3OutMax=[]  SumDOutMin=[]  SumDOutMax=[]  SaturationOutMin=[]  SaturationOutMax=[]  IntegratorContinuousStateAttributes=''  IntegratorStateMustResolveToSignalObject=off  IntegratorRTWStateStorageClass=Auto  FilterContinuousStateAttributes=''  FilterStateMustResolveToSignalObject=off  FilterRTWStateStorageClass=Auto  DifferentiatorICPrevScaledInput=0  DifferentiatorOutMin=[]  DifferentiatorOutMax=[]
  PID Controller1 : simulink/Continuous/PID Controller  Controller=PI  TimeDomain=Continuous-time  SampleTime=-1  IntegratorMethod=Forward Euler  FilterMethod=Forward Euler  Form=Parallel  UseFilter=on  ControllerParametersSource=external  P=1  I=1  D=0  N=100  InitialConditionSource=internal  InitialConditionForIntegrator=0  InitialConditionForFilter=0  ExternalReset=none  LimitOutput=off  UpperSaturationLimit=inf  LowerSaturationLimit=-inf  LinearizeAsGain=on  AntiWindupMode=none  Kb=1  TrackingMode=off  Kt=1  PParamMin=[]  PParamMax=[]  IParamMin=[]  IParamMax=[]  DParamMin=[]  DParamMax=[]  NParamMin=[]  NParamMax=[]  KbParamMin=[]  KbParamMax=[]  KtParamMin=[]  KtParamMax=[]  POutMin=[]  POutMax=[]  IOutMin=[]  IOutMax=[]  DOutMin=[]  DOutMax=[]  NOutMin=[]  NOutMax=[]  KbOutMin=[]  KbOutMax=[]  KtOutMin=[]  KtOutMax=[]  IntegratorOutMin=[]  IntegratorOutMax=[]  FilterOutMin=[]  FilterOutMax=[]  SumOutMin=[]  SumOutMax=[]  SumI1OutMin=[]  SumI1OutMax=[]  SumI2OutMin=[]  SumI2OutMax=[]  SumI3OutMin=[]  SumI3OutMax=[]  SumDOutMin=[]  SumDOutMax=[]  SaturationOutMin=[]  SaturationOutMax=[]  IntegratorContinuousStateAttributes=''  IntegratorStateMustResolveToSignalObject=off  IntegratorRTWStateStorageClass=Auto  FilterContinuousStateAttributes=''  FilterStateMustResolveToSignalObject=off  FilterRTWStateStorageClass=Auto  DifferentiatorICPrevScaledInput=0  DifferentiatorOutMin=[]  DifferentiatorOutMax=[]
  PID Controller2 : simulink/Continuous/PID Controller  Controller=PI  TimeDomain=Continuous-time  SampleTime=-1  IntegratorMethod=Forward Euler  FilterMethod=Forward Euler  Form=Parallel  UseFilter=on  ControllerParametersSource=external  P=1  I=1  D=0  N=100  InitialConditionSource=internal  InitialConditionForIntegrator=0  InitialConditionForFilter=0  ExternalReset=none  LimitOutput=off  UpperSaturationLimit=inf  LowerSaturationLimit=-inf  LinearizeAsGain=on  AntiWindupMode=none  Kb=1  TrackingMode=off  Kt=1  PParamMin=[]  PParamMax=[]  IParamMin=[]  IParamMax=[]  DParamMin=[]  DParamMax=[]  NParamMin=[]  NParamMax=[]  KbParamMin=[]  KbParamMax=[]  KtParamMin=[]  KtParamMax=[]  POutMin=[]  POutMax=[]  IOutMin=[]  IOutMax=[]  DOutMin=[]  DOutMax=[]  NOutMin=[]  NOutMax=[]  KbOutMin=[]  KbOutMax=[]  KtOutMin=[]  KtOutMax=[]  IntegratorOutMin=[]  IntegratorOutMax=[]  FilterOutMin=[]  FilterOutMax=[]  SumOutMin=[]  SumOutMax=[]  SumI1OutMin=[]  SumI1OutMax=[]  SumI2OutMin=[]  SumI2OutMax=[]  SumI3OutMin=[]  SumI3OutMax=[]  SumDOutMin=[]  SumDOutMax=[]  SaturationOutMin=[]  SaturationOutMax=[]  IntegratorContinuousStateAttributes=''  IntegratorStateMustResolveToSignalObject=off  IntegratorRTWStateStorageClass=Auto  FilterContinuousStateAttributes=''  FilterStateMustResolveToSignalObject=off  FilterRTWStateStorageClass=Auto  DifferentiatorICPrevScaledInput=0  DifferentiatorOutMin=[]  DifferentiatorOutMax=[]
  PID Controller4 : simulink/Continuous/PID Controller  Controller=PI  TimeDomain=Continuous-time  SampleTime=-1  IntegratorMethod=Forward Euler  FilterMethod=Forward Euler  Form=Parallel  UseFilter=on  ControllerParametersSource=external  P=2  I=0.5  D=0  N=100  InitialConditionSource=internal  InitialConditionForIntegrator=0  InitialConditionForFilter=0  ExternalReset=none  LimitOutput=off  UpperSaturationLimit=inf  LowerSaturationLimit=-inf  LinearizeAsGain=on  AntiWindupMode=none  Kb=1  TrackingMode=off  Kt=1  PParamMin=[]  PParamMax=[]  IParamMin=[]  IParamMax=[]  DParamMin=[]  DParamMax=[]  NParamMin=[]  NParamMax=[]  KbParamMin=[]  KbParamMax=[]  KtParamMin=[]  KtParamMax=[]  POutMin=[]  POutMax=[]  IOutMin=[]  IOutMax=[]  DOutMin=[]  DOutMax=[]  NOutMin=[]  NOutMax=[]  KbOutMin=[]  KbOutMax=[]  KtOutMin=[]  KtOutMax=[]  IntegratorOutMin=[]  IntegratorOutMax=[]  FilterOutMin=[]  FilterOutMax=[]  SumOutMin=[]  SumOutMax=[]  SumI1OutMin=[]  SumI1OutMax=[]  SumI2OutMin=[]  SumI2OutMax=[]  SumI3OutMin=[]  SumI3OutMax=[]  SumDOutMin=[]  SumDOutMax=[]  SaturationOutMin=[]  SaturationOutMax=[]  IntegratorContinuousStateAttributes=''  IntegratorStateMustResolveToSignalObject=off  IntegratorRTWStateStorageClass=Auto  FilterContinuousStateAttributes=''  FilterStateMustResolveToSignalObject=off  FilterRTWStateStorageClass=Auto  DifferentiatorICPrevScaledInput=0  DifferentiatorOutMin=[]  DifferentiatorOutMax=[]
  Sum : Sum  Inputs=|+-
  Sum1 : Sum  Inputs=-+|
  Sum{2,5..10} (7 alike) : Sum  Inputs=|++
  Sum3 : Sum  Inputs=-+|
  Sum4 : Sum  Inputs=|+-
  Trimmed actuator signals : Display
  Tuning perturbation : Step  Commented=on  Time=20  After=3*pi/180  SampleTime=0
  Tuning perturbation2 : Step  Commented=on  Time=20  After=-3*pi/180  SampleTime=0
  Tuning perturbation3 : Step  Commented=on  Time=20  After=3*pi/180  SampleTime=0
  euler_ref : Constant  Value=[0,0,0]
  Controller output : Outport
  wires:
  euler_ref/1 -> Sum/1
  Demux1/3 -> [psi_error]
  Demux1/2 -> [theta_error]
  Demux1/1 -> [phi_error]
  Sum/1 -> Demux1/1
  Bus Selector/1 -> Sum/2  "<euler>"
  earth_ref/1 -> Demux8/1
  Demux8/1 -> [Xearth_ref]
  Demux8/2 -> [Yearth_ref]
  Demux8/3 -> [Zearth_ref]
  Sum3/1 -> Earth to body/1
  Earth to body/1 -> Demux4/1
  Bus Selector/4 -> Earth to body/2  "<DCM>"
  [Vz_body_ref] -> Mux3/3
  [Vx_body_ref] -> Mux3/1
  [Vy_body_ref] -> Mux3/2
  Demux6/3 -> [vz_error]
  Demux6/2 -> [vy_error]
  Demux6/1 -> [vx_error]
  Sum4/1 -> Demux6/1
  Bus Selector/5 -> Sum4/2, Demux7/1  "<V_b>"
  Demux7/3 -> [vz_b]
  Demux7/2 -> [vy_b]
  Demux7/1 -> [vx_b]
  Mux3/1 -> Sum4/1
  [Zearth_ref] -> Mux1/3
  [Xearth_ref] -> Mux1/1
  [Yearth_ref] -> Mux1/2
  Mux1/1 -> Sum3/2
  Demux4/1 -> [x_error]
  Demux4/2 -> [y_error]
  Demux4/3 -> [z_error]
  Demux5/1 -> [X_earth]
  Demux5/2 -> [Y_earth]
  Demux5/3 -> [Z_earth]
  Bus Selector/3 -> Sum3/1, Demux5/1  "<X_e>"
  [r_error] -> Inner Rate Controller1/3
  [q_error] -> Inner Rate Controller1/2
  [p_error] -> Inner Rate Controller1/1
  Inner Rate Controller1/1 -> Sum2/1
  [r_ref] -> Mux2/3
  [p_ref] -> Mux2/1
  [q_ref] -> Mux2/2
  Mux2/1 -> Sum1/2
  [trimmed_input] -> Sum2/2
  trim_control_input/1 -> [trimmed_input]
  Demux/1 -> [p_error]
  Demux/2 -> [q_error]
  Demux/3 -> [r_error]
  Sum1/1 -> Demux/1
  Bus Selector/2 -> Sum1/1, Demux3/1  "<omega_b>"
  measurements/1 -> Bus Selector/1
  Demux3/1 -> [p]
  Demux3/2 -> [q]
  Demux3/3 -> [r]
  PID Controller/1 -> [p_ref]
  PID Controller1/1 -> [q_ref]
  PID Controller2/1 -> [r_ref]
  [vz_error] -> PID Controller4/1
  PID Controller4/1 -> Gain2/1, Gain1/1, Gain3/1
  Gain1/1 -> Sum7/2
  Gain2/1 -> Sum5/2
  Gain3/1 -> Sum6/2
  Constant4/1 -> PID Controller4/2
  Constant6/1 -> PID Controller4/3
  Sum6/1 -> Mux4/1  "delta_throttle1"
  Demux2/6 -> Mux4/6  "delta_gamma2"
  Demux2/5 -> Mux4/5  "delta_eta2"
  Demux2/3 -> Mux4/3  "delta_gamma1"
  Demux2/2 -> Mux4/2
  Demux2/9 -> Mux4/9  "delta_gamma3"
  Demux2/8 -> Mux4/8  "delta_eta3"
  Mux4/1 -> Trimmed actuator signals/1, Controller output/1
  Sum5/1 -> Mux4/4
  Sum7/1 -> Mux4/7
  Demux2/7 -> Sum7/1
  Demux2/4 -> Sum5/1
  Demux2/1 -> Sum6/1
  Sum2/1 -> Demux2/1
  Constant2/1 -> PID Controller2/2
  Constant1/1 -> PID Controller2/3
  Constant5/1 -> PID Controller1/2
  Constant8/1 -> PID Controller/2
  Constant7/1 -> PID Controller/3
  Constant3/1 -> PID Controller1/3
  Sum8/1 -> PID Controller/1
  [phi_error] -> Sum8/1
  [theta_error] -> Sum9/1
  [psi_error] -> Sum10/1
  Sum10/1 -> PID Controller2/1
  Sum9/1 -> PID Controller1/1
  Tuning perturbation3/1 -> Sum10/2
  Tuning perturbation/1 -> Sum8/2
  Tuning perturbation2/1 -> Sum9/2

== system lib_controller/Controller/4DOF PID Controller/4DOF PI Rate Trimming Controller ==
  note: This block is used to calculate the trimming values for the inner loop rates
  note: INNER LOOP TUNING
  measurements : Inport
  earth_ref : Inport  Port=2
  trim_control_input : Inport  Port=3
  Bus Selector : BusSelector  OutputSignals=euler,euler_dot
  Demux{,1..5} (6 alike) : Demux  Outputs=3
  Euler_dot_ref : Constant  Value=[0 0 0]
  Euler_ref : Constant  Value=[0 0 0]
  Inner Rate Controller : ModelReference  ModelNameDialog=Inner_Rate_Controller  SimulationMode=Normal  ModelReferenceVersion=1.1241  CopyOfModelName=Inner_Rate_Controller
  Sum : Sum  Inputs=|+-
  Sum1 : Sum  Inputs=-+|
  Sum2 : Sum  Inputs=|++
  Controller output : Outport
  wires:
  trim_control_input/1 -> [trimmed_input]
  Demux1/3 -> [psi_error]
  Demux1/2 -> [theta_error]
  Demux1/1 -> [phi_error]
  Demux/1 -> [p_error]
  Demux/2 -> [q_error]
  Demux/3 -> [r_error]
  Sum/1 -> Demux1/1
  Sum1/1 -> Demux/1
  Bus Selector/2 -> Sum1/1, Demux3/1  "<euler_dot>"
  Bus Selector/1 -> Sum/2, Demux2/1  "<euler>"
  measurements/1 -> Bus Selector/1
  Demux2/3 -> [psi]
  Demux2/2 -> [theta]
  Demux2/1 -> [phi]
  Demux3/1 -> [p]
  Demux3/2 -> [q]
  Demux3/3 -> [r]
  Demux4/3 -> [psi_ref]
  Demux4/2 -> [theta_ref]
  Demux4/1 -> [phi_ref]
  Euler_ref/1 -> Demux4/1, Sum/1
  Demux5/1 -> [p_ref]
  Demux5/2 -> [q_ref]
  Demux5/3 -> [r_ref]
  Euler_dot_ref/1 -> Demux5/1, Sum1/2
  [r_error] -> Inner Rate Controller/3
  [p_error] -> Inner Rate Controller/1
  [q_error] -> Inner Rate Controller/2
  Inner Rate Controller/1 -> Sum2/1
  Sum2/1 -> Controller output/1
  [trimmed_input] -> Sum2/2

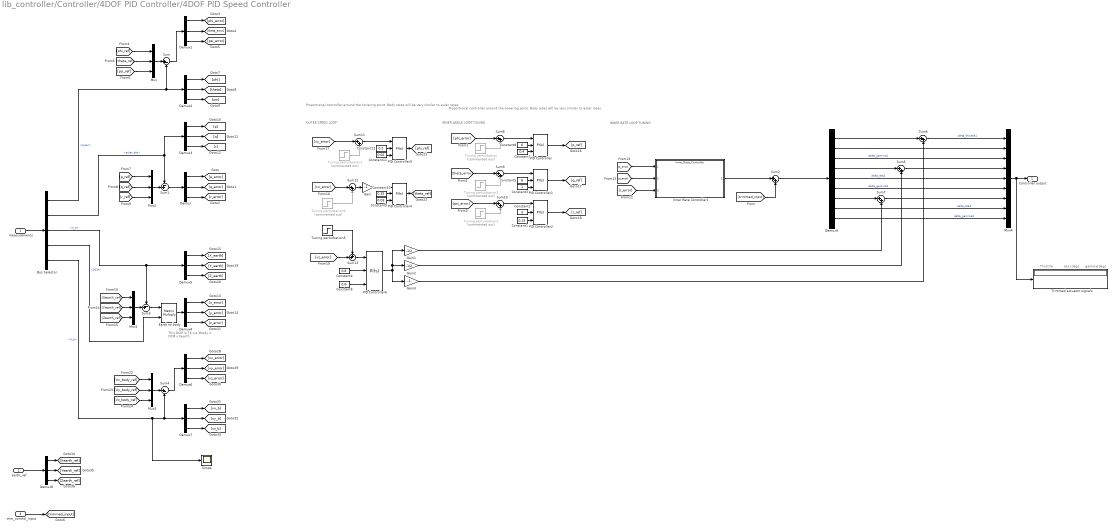
== system lib_controller/Controller/4DOF PID Controller/4DOF PID Speed Controller ==
  note: This DCM is Tb->e
      | Xbody = DCM x Xearth
  note: Proportional controller around the hovering point. Body rates will be very similar to euler rates.
  note: OUTER SPEED LOOP
  note: Throttle
  note: INNER ANGLE LOOP TUNING
  note: INNER RATE LOOP TUNING
  note: Proportional controller around the hovering point. Body rates will be very similar to euler rates.
  note: eta [deg]
  note: gamma[deg]
  measurements : Inport
  earth_ref : Inport  Port=2
  trim_control_input : Inport  Port=3
  Bus Selector : BusSelector  OutputSignals=euler,euler_dot,X_e,DCM,V_b
  Constant1 : Constant  Value=0.15
  Constant10 : Constant  Value=0.35
  Constant11 : Constant  Value=0.02
  Constant12 : Constant  Value=0.2
  Constant2 : Constant  Value=3
  Constant3 : Constant
  Constant4 : Constant  Value=0.8
  Constant5 : Constant  Value=6
  Constant6 : Constant  Value=0.6
  Constant7 : Constant  Value=0.4
  Constant8 : Constant  Value=6
  Constant9 : Constant  Value=0.03
  Demux{,1..8} (9 alike) : Demux  Outputs=3
  Demux9 : Demux  Outputs=9
  Earth to body : Product  Multiplication=Matrix(*)
  Gain : Gain  Gain=-1
  Gain1 : Gain  Gain=-1/2
  Gain2 : Gain  Gain=-1/2
  Gain3 : Gain  Gain=-1
  Inner Rate Controller1 : ModelReference  ModelNameDialog=Inner_Rate_Controller  SimulationMode=Normal  ModelReferenceVersion=1.1241  CopyOfModelName=Inner_Rate_Controller
  Mux{,1..3} (4 alike) : Mux  Inputs=3
  Mux4 : Mux  Inputs=9
  PID Controller{,1..4} (5 alike) : simulink/Continuous/PID Controller  Controller=PI  TimeDomain=Continuous-time  SampleTime=-1  IntegratorMethod=Forward Euler  FilterMethod=Forward Euler  Form=Parallel  UseFilter=on  ControllerParametersSource=external  P=1  I=1  D=0  N=100  InitialConditionSource=internal  InitialConditionForIntegrator=0  InitialConditionForFilter=0  ExternalReset=none  LimitOutput=off  UpperSaturationLimit=inf  LowerSaturationLimit=-inf  LinearizeAsGain=on  AntiWindupMode=none  Kb=1  TrackingMode=off  Kt=1  PParamMin=[]  PParamMax=[]  IParamMin=[]  IParamMax=[]  DParamMin=[]  DParamMax=[]  NParamMin=[]  NParamMax=[]  KbParamMin=[]  KbParamMax=[]  KtParamMin=[]  KtParamMax=[]  POutMin=[]  POutMax=[]  IOutMin=[]  IOutMax=[]  DOutMin=[]  DOutMax=[]  NOutMin=[]  NOutMax=[]  KbOutMin=[]  KbOutMax=[]  KtOutMin=[]  KtOutMax=[]  IntegratorOutMin=[]  IntegratorOutMax=[]  FilterOutMin=[]  FilterOutMax=[]  SumOutMin=[]  SumOutMax=[]  SumI1OutMin=[]  SumI1OutMax=[]  SumI2OutMin=[]  SumI2OutMax=[]  SumI3OutMin=[]  SumI3OutMax=[]  SumDOutMin=[]  SumDOutMax=[]  SaturationOutMin=[]  SaturationOutMax=[]  IntegratorContinuousStateAttributes=''  IntegratorStateMustResolveToSignalObject=off  IntegratorRTWStateStorageClass=Auto  FilterContinuousStateAttributes=''  FilterStateMustResolveToSignalObject=off  FilterRTWStateStorageClass=Auto  DifferentiatorICPrevScaledInput=0  DifferentiatorOutMin=[]  DifferentiatorOutMax=[]
  PID Controller6 : simulink/Continuous/PID Controller  Controller=PI  TimeDomain=Continuous-time  SampleTime=-1  IntegratorMethod=Forward Euler  FilterMethod=Forward Euler  Form=Parallel  UseFilter=on  ControllerParametersSource=external  P=2  I=0.5  D=0  N=100  InitialConditionSource=internal  InitialConditionForIntegrator=0  InitialConditionForFilter=0  ExternalReset=none  LimitOutput=off  UpperSaturationLimit=inf  LowerSaturationLimit=-inf  LinearizeAsGain=on  AntiWindupMode=none  Kb=1  TrackingMode=off  Kt=1  PParamMin=[]  PParamMax=[]  IParamMin=[]  IParamMax=[]  DParamMin=[]  DParamMax=[]  NParamMin=[]  NParamMax=[]  KbParamMin=[]  KbParamMax=[]  KtParamMin=[]  KtParamMax=[]  POutMin=[]  POutMax=[]  IOutMin=[]  IOutMax=[]  DOutMin=[]  DOutMax=[]  NOutMin=[]  NOutMax=[]  KbOutMin=[]  KbOutMax=[]  KtOutMin=[]  KtOutMax=[]  IntegratorOutMin=[]  IntegratorOutMax=[]  FilterOutMin=[]  FilterOutMax=[]  SumOutMin=[]  SumOutMax=[]  SumI1OutMin=[]  SumI1OutMax=[]  SumI2OutMin=[]  SumI2OutMax=[]  SumI3OutMin=[]  SumI3OutMax=[]  SumDOutMin=[]  SumDOutMax=[]  SaturationOutMin=[]  SaturationOutMax=[]  IntegratorContinuousStateAttributes=''  IntegratorStateMustResolveToSignalObject=off  IntegratorRTWStateStorageClass=Auto  FilterContinuousStateAttributes=''  FilterStateMustResolveToSignalObject=off  FilterRTWStateStorageClass=Auto  DifferentiatorICPrevScaledInput=0  DifferentiatorOutMin=[]  DifferentiatorOutMax=[]
  Scope : Scope
      settings: YMin=-1.1  YMax=0.8  SaveName=ScopeData7
  Sum : Sum  Inputs=|+-
  Sum1 : Sum  Inputs=-+|
  Sum{2,5..12} (9 alike) : Sum  Inputs=|++
  Sum13 : Sum  Inputs=++|
  Sum3 : Sum  Inputs=-+|
  Sum4 : Sum  Inputs=|+-
  Trimmed actuator signals : Display
  Tuning perturbation : Step  Commented=on  Time=20  After=3*pi/180  SampleTime=0
  Tuning perturbation1 : Step  Commented=on  Time=20  SampleTime=0
  Tuning perturbation2 : Step  Commented=on  Time=20  After=-3*pi/180  SampleTime=0
  Tuning perturbation3 : Step  Commented=on  Time=20  After=3*pi/180  SampleTime=0
  Tuning perturbation4 : Step  Commented=on  Time=20  SampleTime=0
  Tuning perturbation5 : Step  Time=20  After=-1  SampleTime=0
  Controller output : Outport
  wires:
  Mux/1 -> Sum/1
  Demux3/3 -> [r]
  Demux3/2 -> [q]
  Demux3/1 -> [p]
  Demux2/1 -> [phi]
  Demux2/2 -> [theta]
  Demux2/3 -> [psi]
  measurements/1 -> Bus Selector/1
  Bus Selector/1 -> Demux2/1, Sum/2  "<euler>"
  Bus Selector/2 -> Demux3/1, Sum1/1  "<euler_dot>"
  Sum1/1 -> Demux/1
  Sum/1 -> Demux1/1
  Demux/3 -> [r_error]
  Demux/2 -> [q_error]
  Demux/1 -> [p_error]
  Demux1/1 -> [phi_error]
  Demux1/2 -> [theta_error]
  Demux1/3 -> [psi_error]
  trim_control_input/1 -> [trimmed_input]
  [theta_ref] -> Mux/2
  [phi_ref] -> Mux/1
  [psi_ref] -> Mux/3
  Mux2/1 -> Sum1/2
  [q_ref] -> Mux2/2
  [p_ref] -> Mux2/1
  [r_ref] -> Mux2/3
  Bus Selector/3 -> Demux5/1, Sum3/1  "<X_e>"
  Demux5/3 -> [Z_earth]
  Demux5/2 -> [Y_earth]
  Demux5/1 -> [X_earth]
  Demux4/3 -> [z_error]
  Demux4/2 -> [y_error]
  Demux4/1 -> [x_error]
  Mux1/1 -> Sum3/2
  [Yearth_ref] -> Mux1/2
  [Xearth_ref] -> Mux1/1
  [Zearth_ref] -> Mux1/3
  Mux3/1 -> Sum4/1
  Demux7/1 -> [vx_b]
  Demux7/2 -> [vy_b]
  Demux7/3 -> [vz_b]
  Bus Selector/5 -> Scope/1, Demux7/1, Sum4/2  "<V_b>"
  Sum4/1 -> Demux6/1
  Demux6/1 -> [vx_error]
  Demux6/2 -> [vy_error]
  Demux6/3 -> [vz_error]
  [Vy_body_ref] -> Mux3/2
  [Vx_body_ref] -> Mux3/1
  [Vz_body_ref] -> Mux3/3
  Bus Selector/4 -> Earth to body/2  "<DCM>"
  Earth to body/1 -> Demux4/1
  Sum3/1 -> Earth to body/1
  Demux8/3 -> [Zearth_ref]
  Demux8/2 -> [Yearth_ref]
  Demux8/1 -> [Xearth_ref]
  earth_ref/1 -> Demux8/1
  [r_error] -> Inner Rate Controller1/3
  [q_error] -> Inner Rate Controller1/2
  [p_error] -> Inner Rate Controller1/1
  Inner Rate Controller1/1 -> Sum2/1
  [trimmed_input] -> Sum2/2
  PID Controller/1 -> [p_ref]
  PID Controller1/1 -> [q_ref]
  PID Controller2/1 -> [r_ref]
  PID Controller6/1 -> Gain2/1, Gain1/1, Gain3/1
  Gain1/1 -> Sum7/2
  Gain2/1 -> Sum5/2
  Gain3/1 -> Sum6/2
  Constant4/1 -> PID Controller6/2
  Constant6/1 -> PID Controller6/3
  Sum6/1 -> Mux4/1  "delta_throttle1"
  Demux9/6 -> Mux4/6  "delta_gamma2"
  Demux9/5 -> Mux4/5  "delta_eta2"
  Demux9/3 -> Mux4/3  "delta_gamma1"
  Demux9/2 -> Mux4/2
  Demux9/9 -> Mux4/9  "delta_gamma3"
  Demux9/8 -> Mux4/8  "delta_eta3"
  Mux4/1 -> Trimmed actuator signals/1, Controller output/1
  Sum5/1 -> Mux4/4
  Sum7/1 -> Mux4/7
  Demux9/7 -> Sum7/1
  Demux9/4 -> Sum5/1
  Demux9/1 -> Sum6/1
  Sum2/1 -> Demux9/1
  Constant2/1 -> PID Controller2/2
  Constant1/1 -> PID Controller2/3
  Constant5/1 -> PID Controller1/2
  Constant8/1 -> PID Controller/2
  Constant7/1 -> PID Controller/3
  Constant3/1 -> PID Controller1/3
  Sum8/1 -> PID Controller/1
  [phi_error] -> Sum8/1
  [theta_error] -> Sum9/1
  [psi_error] -> Sum10/1
  Sum10/1 -> PID Controller2/1
  Sum9/1 -> PID Controller1/1
  Tuning perturbation3/1 -> Sum10/2
  Tuning perturbation/1 -> Sum8/2
  Tuning perturbation2/1 -> Sum9/2
  PID Controller3/1 -> [phi_ref]
  PID Controller4/1 -> [theta_ref]
  Constant10/1 -> PID Controller4/2
  Constant12/1 -> PID Controller3/2
  Constant11/1 -> PID Controller3/3
  Constant9/1 -> PID Controller4/3
  Sum11/1 -> PID Controller3/1
  [vy_error] -> Sum11/1
  [vx_error] -> Sum12/1
  Sum12/1 -> Gain/1
  Tuning perturbation1/1 -> Sum11/2
  Tuning perturbation4/1 -> Sum12/2
  Gain/1 -> PID Controller4/1
  Tuning perturbation5/1 -> Sum13/1
  [vz_error] -> Sum13/2
  Sum13/1 -> PID Controller6/1
